simulink library "ddm"  (R2021b)
settings: Solver=VariableStepAuto  StartTime=0.0  StopTime=10.0  RelTol=1e-3
undefined symbols (not defined in the file): ADDM_FrTMTqDev_X_Nm, ADDM_RrTMTqDev_X_Nm, ENUM_ADASACCSTA_ERROR, ENUM_ADASACCSTA_OFF, ENUM_ADASACCSTA_STANDBY, ENUM_ALLOWMOV_ALLOWREADY, ENUM_APS, ENUM_BRKSTA_ERROR, ENUM_BRKSTA_OFF, ENUM_BRKSTA_ON, ENUM_BRKSW_INVALID, ENUM_BRKSW_OFF, ENUM_BRKSW_ON, ENUM_CHGPREACTERRSTA_OBCPRE, ENUM_DCDCFAULTSTA_ANYFAULTLV1, ENUM_DCDCFAULTSTA_ANYFAULTLV2, ENUM_DRIVETRAIN_AWD, ENUM_DRIVETRAIN_FWD, ENUM_DRIVETRAIN_RWD, ENUM_EDUDRTSTA_NORMAL, ENUM_EPBERROR_FAILED, ENUM_EPBSTA_APPLIED, ENUM_EPBSTA_RELEASED, ENUM_ESCAPSSta_APSUNAVAILABLE, ENUM_GEARACTUALPOSN_INVALID, ENUM_GEARACTUALPOSN_P, ENUM_HVBATTREADYPRE_READY, ENUM_HWRESETSTA_HWRESETING, ENUM_MCUWARN_LV0, ENUM_MCUWARN_LV1, ENUM_MCUWARN_LV2, ENUM_MCUWARN_LV3, ENUM_MCUWARN_NOERROR, ENUM_OBCFAULTSTA_ANYFAULT, ENUM_PAS_R2F2, ENUM_PDFAULT_BATTPDFAIL, ENUM_PDFAULT_DCDCDISABLE, ENUM_PDFAULT_MCUDISABLE, ENUM_PDFAULT_MCUDISCHRG, ENUM_POWERSTA_OFF, ENUM_POWERSTA_ON, ENUM_POWERSTA_READY, ENUM_POWERSTA_STANDBY, ENUM_PRESSINDI_LOW, ENUM_PUFAULT_BATTUPFAIL, ENUM_PUFAULT_DCDCENABLEFAIL, ENUM_PUFAULT_PRECHRGCHKFAIL, ENUM_PUFAULT_SAFETYCHKFAIL, ENUM_PWRSTASW_OFF, ENUM_PWRSTASW_OFFA, ENUM_PWRSTASW_OFFCHVCHRG, ENUM_PWRSTASW_OFFCLVCHRG, ENUM_PWRSTASW_ON, ENUM_PWRSTASW_ONHVCHRG, ENUM_PWRSTASW_READY, ENUM_PWRSTASW_STANDBY, ENUM_RAPSErrWarnSta_NORMAL, ENUM_RAPSErrWarnSta_RAPSERRLV1, ENUM_SHIFTCOMMAND_P, ENUM_SHIFTERERRSTA_PBUTTONFAILURE ... (+471)
libraries: hcu_lib x540, simulink x3
(part 20 of 26)

== system ddm/DDM/DDM/PMM/Fault level/Fault level 4 subsystem error1 ==
  note: Test Pass Criteria
  note: Release Condition After Failure Decision
  note: Diagnostics and Fault Handling
  note: Test Detection Criteria
  task_time_s : Inport
  VPMM_PowerSta_enum : Inport  Port=2
  VPMM_PwrStaSW_enum : Inport  Port=3
  VDDM_C3BMS6LCCFS_flg : Inport  Port=4
  VINP_BMSWarn7_flg : Inport  Port=5
  VINP_BMSWarn8_flg : Inport  Port=6
  DTC_clear_request : Inport  Port=7
  No_CAN3_BUS_OFF : Inport  Port=8
  VDDM_C3BMS6RCCFS_flg : Inport  Port=9
  VDDM_C3BMS6CSCFS_flg : Inport  Port=10
  ZoneDrMalfunLevel_enum : Inport  Port=11
  No_CAN4_BUS_OFF : Inport  Port=12
  VDDM_DrVCUNoComCFS_flg : Inport  Port=13
  ZoneFrMalfunLevel_enum : Inport  Port=14
  VDDM_FrVCUNoComCFS_flg : Inport  Port=15
  AND2 : Logic  Inputs=5  AllPortsSameDT=off  OutDataTypeStr=boolean
  AND5 : Logic  Inputs=3  AllPortsSameDT=off  OutDataTypeStr=boolean
  AND6 : Logic  Inputs=3  AllPortsSameDT=off  OutDataTypeStr=boolean
  Constant1 : Constant  Value=ENUM_PWRSTASW_OFF
  Constant12 : Constant  Value=KDDM_FaultLvDiagnosisOffSW_flg
  Constant14 : Constant  Value=ZERO_INT
  Constant18 : Constant  Value=KDDM_Lv4ErrPassTO_s
  Constant19 : Constant  Value=ENUM_POWERSTA_OFF
  Constant2 : Constant  Value=TRUE
  Constant22 : Constant  Value=FALSE
  Constant24 : Constant  Value=TRUE
  Constant25 : Constant  Value=FALSE
  Constant26 : Constant  Value=ENUM_PWRSTASW_OFF
  Constant27 : Constant  Value=FALSE
  Constant3 : Constant  Value=KDDM_Lv4ErrDetTO_s
  Constant4 : Constant  Value=KDDM_Lv4ErrPassTO_s
  Constant40 : Constant  Value=KDDM_Lv4ErrDTC_cnt
  Constant5 : Constant  Value=KDDM_Lv4ErrDTC_cnt
  Constant6 : Constant  Value=ENUM_ZONEMALFUNLV_4TH
  Constant7 : Constant  Value=ENUM_ZONEMALFUNLV_4TH
  DTC_Couter : hcu_lib/Basic_Blocks/DTC_Couter
  DTC_Info : hcu_lib/Basic_Blocks/DTC_Info
  Delay : Delay  DelayLength=1
  Equal : RelationalOperator  Operator=~=  OutDataTypeStr=boolean  RndMeth=Simplest
  Equal1 : RelationalOperator  Operator===  OutDataTypeStr=boolean  RndMeth=Simplest
  Equal2 : RelationalOperator  Operator=~=  OutDataTypeStr=boolean  RndMeth=Simplest
  Equal3 : RelationalOperator  OutDataTypeStr=boolean  RndMeth=Simplest
  Equal4 : RelationalOperator  Operator===  OutDataTypeStr=boolean  RndMeth=Simplest
  Equal8 : RelationalOperator  Operator===  OutDataTypeStr=boolean  RndMeth=Simplest
  Logical Operator21 : Logic  AllPortsSameDT=off  OutDataTypeStr=boolean
  Logical Operator6 : Logic  Operator=NOT  AllPortsSameDT=off  OutDataTypeStr=boolean
  Logical Operator8 : Logic  Operator=OR  Inputs=4  AllPortsSameDT=off  OutDataTypeStr=boolean
  NOT{,17..19,26,28} (6 alike) : Logic  Operator=NOT  AllPortsSameDT=off  OutDataTypeStr=boolean
  OR : Logic  Operator=OR  Inputs=3  AllPortsSameDT=off  OutDataTypeStr=boolean
  OR1 : Logic  Operator=OR  AllPortsSameDT=off  OutDataTypeStr=boolean
  OR2 : Logic  Operator=OR  Inputs=3  AllPortsSameDT=off  OutDataTypeStr=boolean
  Relational Operator : RelationalOperator  Operator=>  OutDataTypeStr=boolean  RndMeth=Simplest
  Switch{1,4..5,9} (4 alike) : Switch  Criteria=u2 ~= 0
  Terminator : Terminator
  Test Detection Criteria : hcu_lib/Basic_Blocks/Test Detection Criteria
  Timer1 : hcu_lib/Basic_Blocks/Timer
  VDDM_Lv4ErrCFS_flg : Outport
  VDDM_Lv4ErrDTC_raw32 : Outport  Port=2
  wires:
  Switch9/1 -> Test Detection Criteria/1
  Constant22/1 -> Switch9/1
  [VDDM_Lv4ErrCFSRls_flg] -> Switch9/2
  DTC_Info/1 -> VDDM_Lv4ErrDTC_raw32/1  "VDDM_Lv4ErrDTC_raw32"
  [VDDM_Lv4ErrPass_flg] -> DTC_Info/2
  [VDDM_Lv4ErrDet_flg] -> DTC_Info/1
  [VDDM_Lv4ErrCFS_flg] -> DTC_Info/3
  [DTC_clear_request] -> DTC_Info/4
  VDDM_FrVCUNoComCFS_flg/1 -> [VDDM_FrVCUNoComCFS_flg]
  ZoneFrMalfunLevel_enum/1 -> [ZoneFrMalfunLevel_enum]
  VDDM_DrVCUNoComCFS_flg/1 -> [VDDM_DrVCUNoComCFS_flg]
  No_CAN4_BUS_OFF/1 -> [No_CAN4_BUS_OFF]
  ZoneDrMalfunLevel_enum/1 -> [ZoneDrMalfunLevel_enum]
  VDDM_C3BMS6CSCFS_flg/1 -> [VDDM_C3BMS6CSCFS_flg]
  VDDM_C3BMS6RCCFS_flg/1 -> [VDDM_C3BMS6RCCFS_flg]
  [VDDM_Lv4ErrCFS_flg] -> VDDM_Lv4ErrCFS_flg/1
  Equal2/1 -> Switch1/2
  [VDDM_BMSFaultLv4_flg] -> OR2/1
  OR2/1 -> Switch1/1
  [VDDM_ZoneFrFaultLv4_flg] -> OR2/3
  Constant1/1 -> Equal2/2
  [VDDM_ZoneDrFaultLv4_flg] -> OR2/2
  [VPMM_PwrStaSW_enum] -> Equal2/1
  Constant2/1 -> Switch1/3
  OR/1 -> Switch5/1
  [VDDM_BMSFaultLv4_flg] -> OR/1
  [VDDM_ZoneDrFaultLv4_flg] -> OR/2
  [VDDM_ZoneFrFaultLv4_flg] -> OR/3
  AND5/1 -> [VDDM_ZoneDrFaultLv4_flg]  "VDDM_ZoneDrFaultLv4_flg"
  [VINP_BMSWarn7_flg] -> OR1/1
  [VDDM_C3BMS6CSCFS_flg] -> NOT19/1
  NOT19/1 -> AND2/5
  Constant7/1 -> Equal8/2
  NOT18/1 -> AND2/4
  [VINP_BMSWarn8_flg] -> OR1/2
  [No_CAN4_BUS_OFF] -> AND5/2
  [ZoneFrMalfunLevel_enum] -> Equal8/1
  Equal8/1 -> AND6/1
  NOT26/1 -> AND5/3
  [ZoneDrMalfunLevel_enum] -> Equal1/1
  OR1/1 -> AND2/1
  [VDDM_DrVCUNoComCFS_flg] -> NOT26/1
  AND2/1 -> [VDDM_BMSFaultLv4_flg]  "VDDM_BMSFaultLv4_flg"
  NOT17/1 -> AND2/3
  Constant6/1 -> Equal1/2
  Equal1/1 -> AND5/1
  [No_CAN4_BUS_OFF] -> AND6/2
  AND6/1 -> [VDDM_ZoneFrFaultLv4_flg]  "VDDM_ZoneFrFaultLv4_flg"
  [VDDM_FrVCUNoComCFS_flg] -> NOT28/1
  NOT28/1 -> AND6/3
  [VDDM_C3BMS6RCCFS_flg] -> NOT18/1
  [No_CAN3_BUS_OFF] -> AND2/2
  [VDDM_C3BMS6LCCFS_flg] -> NOT17/1
  Constant14/1 -> Relational Operator/2
  [VDDM_Lv4ErrCFSRls_flg] -> DTC_Couter/2
  [VDDM_Lv4ErrDet_flg] -> DTC_Couter/1
  [VDDM_Lv4ErrPass_flg] -> Logical Operator21/1
  Logical Operator21/1 -> Logical Operator8/3
  [VDDM_Lv4ErrCFS_flg] -> Delay/1
  Delay/1 -> NOT/1
  NOT/1 -> Logical Operator21/2
  Constant12/1 -> Logical Operator8/4
  Switch5/1 -> Switch9/3
  Constant3/1 -> Test Detection Criteria/4
  [task_time_s] -> Timer1/3
  No_CAN3_BUS_OFF/1 -> [No_CAN3_BUS_OFF]
  DTC_clear_request/1 -> [DTC_clear_request]
  [VPMM_PwrStaSW_enum] -> Equal/1
  [VPMM_PowerSta_enum] -> Equal4/1
  Constant4/1 -> Timer1/4
  Constant19/1 -> Equal4/2
  Constant25/1 -> Switch4/3
  Test Detection Criteria/1 -> [VDDM_Lv4ErrDet_flg]  "VDDM_Lv4ErrDet_flg"
  Constant27/1 -> Switch5/3
  Switch4/1 -> [VDDM_Lv4ErrCFSRls_flg]  "VDDM_Lv4ErrCFSRls_flg"
  Logical Operator8/1 -> Switch4/2
  Switch1/1 -> Timer1/2, Logical Operator6/1
  Equal/1 -> Switch5/2
  Constant24/1 -> Switch4/1
  Relational Operator/1 -> Terminator/1  "VDDM_Lv4ErrDFS_flg"
  DTC_Couter/1 -> [VDDM_Lv4ErrCFS_flg]  "VDDM_Lv4ErrCFS_flg"
  Constant18/1 -> Equal3/2
  Constant26/1 -> Equal/2
  Timer1/1 -> Equal3/1
  [DTC_clear_request] -> Logical Operator8/2
  Equal4/1 -> Logical Operator8/1
  Constant40/1 -> Test Detection Criteria/3
  DTC_Couter/2 -> Relational Operator/1  "VDDM_Lv4ErrDTC_cnt"
  [task_time_s] -> Test Detection Criteria/2
  Logical Operator6/1 -> Timer1/1
  Constant5/1 -> DTC_Couter/3
  Equal3/1 -> [VDDM_Lv4ErrPass_flg]  "VDDM_Lv4ErrPass_flg"
  VDDM_C3BMS6LCCFS_flg/1 -> [VDDM_C3BMS6LCCFS_flg]
  VINP_BMSWarn7_flg/1 -> [VINP_BMSWarn7_flg]
  task_time_s/1 -> [task_time_s]
  VPMM_PwrStaSW_enum/1 -> [VPMM_PwrStaSW_enum]
  VPMM_PowerSta_enum/1 -> [VPMM_PowerSta_enum]
  VINP_BMSWarn8_flg/1 -> [VINP_BMSWarn8_flg]

== system ddm/DDM/DDM/PMM/LV/Initial LV battery voltage too low ==
  note: Test Detection Criteria
  note: Test Pass Criteria
  note: Release Condition After Decision
  note: Diagnostics and Fault Handling
  task_time_s : Inport
  VPMM_PowerSta_enum : Inport  Port=2
  VPMM_PwrStaSW_enum : Inport  Port=3
  VDDM_AuxBatVolt_V : Inport  Port=4
  VINP_CANMsgValidBMS5_flg : Inport  Port=5
  DTC_clear_request : Inport  Port=6
  Constant1 : Constant  Value=ENUM_PWRSTASW_OFF
  Constant12 : Constant  Value=ENUM_POWERSTA_STANDBY
  Constant13 : Constant  Value=ZERO_INT
  Constant17 : Constant  Value=KDDM_IniLVLoDTC_cnt
  Constant2 : Constant  Value=ENUM_PWRSTASW_OFF
  Constant22 : Constant  Value=KDDM_IniLVLoDetTO_s
  Constant23 : Constant  Value=FALSE
  Constant26 : Constant  Value=ENUM_PWRSTASW_STANDBY
  Constant27 : Constant  Value=FALSE
  Constant28 : Constant  Value=KDDM_IniLVLoPassTO_s
  Constant29 : Constant  Value=KDDM_IniLVLoPassTO_s
  Constant3 : Constant  Value=ENUM_PWRSTASW_STANDBY
  Constant30 : Constant  Value=KDDM_IniLVLoDTC_cnt
  Constant32 : Constant  Value=KDDM_LVDiagnosisOffSW_flg
  Constant33 : Constant  Value=ENUM_POWERSTA_OFF
  Constant34 : Constant  Value=KDDM_IniLVLoThd_mv
  Constant4 : Constant  Value=FALSE
  Constant5 : Constant  Value=KDDM_IniLVLoThd_mv
  DTC_Couter1 : hcu_lib/Basic_Blocks/DTC_Couter
  DTC_Info : hcu_lib/Basic_Blocks/DTC_Info
  Equal{1..2,4,11..12,14} (6 alike) : RelationalOperator  Operator===  OutDataTypeStr=boolean  RndMeth=Simplest
  Equal10 : RelationalOperator  OutDataTypeStr=boolean  RndMeth=Simplest
  Equal13 : RelationalOperator  Operator=<=  OutDataTypeStr=boolean  RndMeth=Simplest
  Equal3 : RelationalOperator  Operator=<=  OutDataTypeStr=boolean  RndMeth=Simplest
  Gain1 : Gain  Gain=1000
  Gain3 : Gain  Gain=1000
  Logical Operator : Logic  Operator=OR  AllPortsSameDT=off  OutDataTypeStr=boolean
  Logical Operator1 : Logic  Operator=OR  AllPortsSameDT=off  OutDataTypeStr=boolean
  Logical Operator14 : Logic  Operator=OR  Inputs=4  AllPortsSameDT=off  OutDataTypeStr=boolean
  Logical Operator16 : Logic  AllPortsSameDT=off  OutDataTypeStr=boolean
  Logical Operator17 : Logic  Operator=NOT  AllPortsSameDT=off  OutDataTypeStr=boolean
  Logical Operator2 : Logic  AllPortsSameDT=off  OutDataTypeStr=boolean
  Logical Operator9 : Logic  AllPortsSameDT=off  OutDataTypeStr=boolean
  Relational Operator1 : RelationalOperator  Operator=>  OutDataTypeStr=boolean  RndMeth=Simplest
  Switch1 : Switch  Criteria=u2 ~= 0
  Switch2 : Switch  Criteria=u2 ~= 0
  Switch7 : Switch  Criteria=u2 ~= 0
  Terminator : Terminator
  Test Detection Criteria1 : hcu_lib/Basic_Blocks/Test Detection Criteria
  Timer2 : hcu_lib/Basic_Blocks/Timer
  Unit Delay1 : UnitDelay  SampleTime=-1  HasFrameUpgradeWarning=on
  VDDM_IniLVLoDTC_raw32 : Outport
  VDDM_IniLVLoCFS_flg : Outport  Port=2
  wires:
  [VDDM_IniLVLoCFS_flg] -> VDDM_IniLVLoCFS_flg/1
  [VDDM_IniLVLoPass_flg] -> Logical Operator14/3
  Logical Operator9/1 -> Switch1/2
  Constant26/1 -> Equal14/1
  Equal13/1 -> Switch1/1
  Gain3/1 -> Equal13/1
  [VDDM_AuxBatVolt_V] -> Gain3/1
  Constant34/1 -> Equal13/2
  DTC_Couter1/2 -> Relational Operator1/1  "VDDM_IniLVLoDTC_cnt"
  Constant28/1 -> Timer2/4
  DTC_Couter1/1 -> [VDDM_IniLVLoCFS_flg]  "VDDM_IniLVLoCFS_flg"
  [VDDM_IniLVLoDet_flg] -> DTC_Couter1/1
  Logical Operator16/1 -> Logical Operator14/1
  Unit Delay1/1 -> Equal11/1
  [DTC_clear_request] -> Logical Operator14/2
  Constant33/1 -> Equal11/2
  Equal11/1 -> Logical Operator16/1
  Test Detection Criteria1/1 -> [VDDM_IniLVLoDet_flg]  "VDDM_IniLVLoDet_flg"
  [VPMM_PowerSta_enum] -> Equal12/1
  Switch7/1 -> Test Detection Criteria1/1
  Constant32/1 -> Logical Operator14/4
  Constant12/1 -> Equal12/2
  [task_time_s] -> Timer2/3
  Logical Operator14/1 -> [VDDM_IniLVLoCFSRls_flg]  "VDDM_IniLVLoCFSRls_flg"
  Constant17/1 -> Test Detection Criteria1/3
  [VPMM_PowerSta_enum] -> Unit Delay1/1
  Relational Operator1/1 -> Terminator/1  "VDDM_IniLVLoDFS_flg"
  Equal12/1 -> Logical Operator16/2
  [task_time_s] -> Test Detection Criteria1/2
  Switch1/1 -> Switch7/3
  Constant30/1 -> DTC_Couter1/3
  Equal10/1 -> [VDDM_IniLVLoPass_flg]  "VDDM_IniLVLoPass_flg"
  [VDDM_IniLVLoCFSRls_flg] -> Switch7/2
  Constant23/1 -> Switch7/1
  Constant22/1 -> Test Detection Criteria1/4
  Constant29/1 -> Equal10/2
  Switch2/1 -> Logical Operator17/1, Timer2/2
  Timer2/1 -> Equal10/1
  Constant27/1 -> Switch1/3
  Logical Operator17/1 -> Timer2/1
  [VDDM_IniLVLoCFSRls_flg] -> DTC_Couter1/2
  Constant13/1 -> Relational Operator1/2
  task_time_s/1 -> [task_time_s]
  VDDM_AuxBatVolt_V/1 -> [VDDM_AuxBatVolt_V]
  VPMM_PwrStaSW_enum/1 -> [VPMM_PwrStaSW_enum]
  VPMM_PowerSta_enum/1 -> [VPMM_PowerSta_enum]
  DTC_clear_request/1 -> [DTC_clear_request]
  VINP_CANMsgValidBMS5_flg/1 -> [VINP_CANMsgValidBMS5_flg]
  DTC_Info/1 -> VDDM_IniLVLoDTC_raw32/1  "VDDM_IniLVLoDTC_raw32"
  [VDDM_IniLVLoPass_flg] -> DTC_Info/2
  [VDDM_IniLVLoCFS_flg] -> DTC_Info/3
  [VDDM_IniLVLoDet_flg] -> DTC_Info/1
  [DTC_clear_request] -> DTC_Info/4
  [VINP_CANMsgValidBMS5_flg] -> Logical Operator9/2
  Constant1/1 -> Equal1/2
  Constant5/1 -> Equal3/2
  Logical Operator2/1 -> Switch2/2
  [VDDM_AuxBatVolt_V] -> Gain1/1
  Constant4/1 -> Switch2/3
  Equal3/1 -> Switch2/1
  Gain1/1 -> Equal3/1
  Logical Operator/1 -> Logical Operator9/1
  Equal14/1 -> Logical Operator/1
  Equal1/1 -> Logical Operator/2
  [VPMM_PwrStaSW_enum] -> Equal14/2, Equal1/1
  Equal4/1 -> Logical Operator1/1
  Constant2/1 -> Equal2/2
  Constant3/1 -> Equal4/1
  Logical Operator1/1 -> Logical Operator2/1
  [VPMM_PwrStaSW_enum] -> Equal4/2, Equal2/1
  Equal2/1 -> Logical Operator1/2
  [VINP_CANMsgValidBMS5_flg] -> Logical Operator2/2

== system ddm/DDM/DDM/PMM/LV/LV analog input error ==
  note: Diagnostics and Fault Handling
  note: Release Condition After Decision
  note: Test Pass Criteria
  note: Test Detection Criteria
  task_time_s : Inport
  VPMM_PowerSta_enum : Inport  Port=2
  VINP_LVBattDet12V_V : Inport  Port=3
  VINP_CANMsgValidBMS5_flg : Inport  Port=4
  DTC_clear_request : Inport  Port=5
  VDDM_AuxBattVolV_V : Inport  Port=6
  VINP_VehicleType_enum : Inport  Port=7
  Abs : Abs
  Abs1 : Abs
  Add : Sum  Inputs=-+
  Add1 : Sum  Inputs=-+
  Constant : Constant  Value=eps
  Constant1 : Constant  Value=eps
  Constant12 : Constant  Value=ENUM_POWERSTA_STANDBY
  Constant13 : Constant  Value=ZERO_INT
  Constant17 : Constant  Value=KDDM_LVInErrDTC_cnt
  Constant2 : Constant  Value=FALSE
  Constant22 : Constant  Value=KDDM_LVInErrDetTO_s
  Constant23 : Constant  Value=FALSE
  Constant27 : Constant  Value=FALSE
  Constant28 : Constant  Value=KDDM_LVInErrPassTO_s
  Constant3 : Constant  Value=KDDM_LVInErr_pct
  Constant30 : Constant  Value=KDDM_LVInErrDTC_cnt
  Constant32 : Constant  Value=KDDM_LVDiagnosisOffSW_flg
  Constant33 : Constant  Value=ENUM_POWERSTA_OFF
  Constant34 : Constant  Value=KDDM_LVInErr_pct
  Constant4 : Constant  Value=KDDM_LVInErrPassTO_s
  Constant5 : Constant  Value=ENUM_VEHICLETYPE_D31L24
  Constant6 : Constant  Value=ENUM_VEHICLETYPE_D31L24
  DTC_Couter1 : hcu_lib/Basic_Blocks/DTC_Couter
  DTC_Info : hcu_lib/Basic_Blocks/DTC_Info
  Divide : Product  Inputs=*/
  Divide1 : Product  Inputs=*/
  Equal1 : RelationalOperator  OutDataTypeStr=boolean  RndMeth=Simplest
  Equal10 : RelationalOperator  OutDataTypeStr=boolean  RndMeth=Simplest
  Equal11 : RelationalOperator  Operator===  OutDataTypeStr=boolean  RndMeth=Simplest
  Equal12 : RelationalOperator  Operator===  OutDataTypeStr=boolean  RndMeth=Simplest
  Equal13 : RelationalOperator  OutDataTypeStr=boolean  RndMeth=Simplest
  Gain : Gain  Gain=100  OutDataTypeStr=single
  Gain1 : Gain  Gain=100  OutDataTypeStr=single
  Logical Operator : Logic  AllPortsSameDT=off  OutDataTypeStr=boolean
  Logical Operator1 : Logic  AllPortsSameDT=off  OutDataTypeStr=boolean
  Logical Operator14 : Logic  Operator=OR  Inputs=4  AllPortsSameDT=off  OutDataTypeStr=boolean
  Logical Operator16 : Logic  AllPortsSameDT=off  OutDataTypeStr=boolean
  Logical Operator17 : Logic  Operator=NOT  AllPortsSameDT=off  OutDataTypeStr=boolean
  Max : MinMax  Function=max  Inputs=2
  Max1 : MinMax  Function=max  Inputs=2
  Relational Operator : RelationalOperator  Operator=~=  OutDataTypeStr=boolean  RndMeth=Simplest
  Relational Operator1 : RelationalOperator  Operator=>  OutDataTypeStr=boolean  RndMeth=Simplest
  Relational Operator2 : RelationalOperator  Operator=~=  OutDataTypeStr=boolean  RndMeth=Simplest
  Switch1 : Switch  Criteria=u2 ~= 0
  Switch2 : Switch  Criteria=u2 ~= 0
  Switch7 : Switch  Criteria=u2 ~= 0
  Terminator : Terminator
  Test Detection Criteria1 : hcu_lib/Basic_Blocks/Test Detection Criteria
  Timer2 : hcu_lib/Basic_Blocks/Timer
  Unit Delay1 : UnitDelay  SampleTime=-1  HasFrameUpgradeWarning=on
  VDDM_LVInErrDTC_raw32 : Outport
  VDDM_LVInErrCFS_flg : Outport  Port=2
  wires:
  [VDDM_LVInErrCFS_flg] -> VDDM_LVInErrCFS_flg/1
  Constant2/1 -> Switch2/3
  [VDDM_AuxBattVolV_V] -> Add1/1
  Constant3/1 -> Equal1/2
  Equal1/1 -> Switch2/1
  [VINP_LVBattDet12V_V] -> Add1/2, Max1/1
  Gain1/1 -> Equal1/1
  Add1/1 -> Divide1/1
  Divide1/1 -> Abs1/1
  Abs1/1 -> Gain1/1
  Constant1/1 -> Max1/2
  Max1/1 -> Divide1/2
  Max/1 -> Divide/2
  Add/1 -> Divide/1
  Constant/1 -> Max/2
  [VINP_LVBattDet12V_V] -> Add/2, Max/1
  [VDDM_AuxBattVolV_V] -> Add/1
  Abs/1 -> Gain/1
  Divide/1 -> Abs/1
  VDDM_AuxBattVolV_V/1 -> [VDDM_AuxBattVolV_V]
  VPMM_PowerSta_enum/1 -> [VPMM_PowerSta_enum]
  VINP_LVBattDet12V_V/1 -> [VINP_LVBattDet12V_V]
  VINP_CANMsgValidBMS5_flg/1 -> [VINP_CANMsgValidBMS5_flg]
  [DTC_clear_request] -> DTC_Info/4
  DTC_clear_request/1 -> [DTC_clear_request]
  [VDDM_LVInErrCFS_flg] -> DTC_Info/3
  task_time_s/1 -> [task_time_s]
  DTC_Info/1 -> VDDM_LVInErrDTC_raw32/1  "VDDM_LVInErrDTC_raw32"
  [VDDM_LVInErrDet_flg] -> DTC_Info/1
  [VDDM_LVInErrPass_flg] -> DTC_Info/2
  Equal10/1 -> [VDDM_LVInErrPass_flg]  "VDDM_LVInErrPass_flg"
  Constant23/1 -> Switch7/1
  Constant13/1 -> Relational Operator1/2
  [VDDM_LVInErrCFSRls_flg] -> Switch7/2
  Constant34/1 -> Equal13/2
  DTC_Couter1/1 -> [VDDM_LVInErrCFS_flg]  "VDDM_LVInErrCFS_flg"
  Equal12/1 -> Logical Operator16/2
  [VDDM_LVInErrCFSRls_flg] -> DTC_Couter1/2
  [VPMM_PowerSta_enum] -> Equal12/1
  Constant12/1 -> Equal12/2
  Switch7/1 -> Test Detection Criteria1/1
  Gain/1 -> Equal13/1
  Constant33/1 -> Equal11/2
  [task_time_s] -> Timer2/3
  Constant30/1 -> DTC_Couter1/3
  Relational Operator1/1 -> Terminator/1  "VDDM_LVInErrDFS_flg"
  Constant22/1 -> Test Detection Criteria1/4
  Logical Operator14/1 -> [VDDM_LVInErrCFSRls_flg]  "VDDM_LVInErrCFSRls_flg"
  Constant27/1 -> Switch1/3
  [VDDM_LVInErrPass_flg] -> Logical Operator14/3
  [VPMM_PowerSta_enum] -> Unit Delay1/1
  Constant17/1 -> Test Detection Criteria1/3
  Unit Delay1/1 -> Equal11/1
  Constant4/1 -> Equal10/2
  Equal11/1 -> Logical Operator16/1
  [DTC_clear_request] -> Logical Operator14/2
  Equal13/1 -> Switch1/1
  [VDDM_LVInErrDet_flg] -> DTC_Couter1/1
  Logical Operator17/1 -> Timer2/1
  DTC_Couter1/2 -> Relational Operator1/1  "VDDM_LVInErrDTC_cnt"
  Logical Operator16/1 -> Logical Operator14/1
  Timer2/1 -> Equal10/1
  Test Detection Criteria1/1 -> [VDDM_LVInErrDet_flg]  "VDDM_LVInErrDet_flg"
  Switch1/1 -> Switch7/3
  Constant28/1 -> Timer2/4
  Switch2/1 -> Logical Operator17/1, Timer2/2
  Constant32/1 -> Logical Operator14/4
  [task_time_s] -> Test Detection Criteria1/2
  VINP_VehicleType_enum/1 -> [VINP_VehicleType_enum]
  [VINP_CANMsgValidBMS5_flg] -> Logical Operator/1
  Logical Operator/1 -> Switch1/2
  Relational Operator/1 -> Logical Operator/2
  [VINP_VehicleType_enum] -> Relational Operator/1
  Constant5/1 -> Relational Operator/2
  [VINP_CANMsgValidBMS5_flg] -> Logical Operator1/1
  [VINP_VehicleType_enum] -> Relational Operator2/1
  Constant6/1 -> Relational Operator2/2
  Relational Operator2/1 -> Logical Operator1/2
  Logical Operator1/1 -> Switch2/2

== system ddm/DDM/DDM/PMM/LV/LV power supply voltage too high ==
  note: Release Condition After Decision
  note: Test Detection Criteria
  note: Test Pass Criteria
  note: Diagnostics and Fault Handling
  task_time_s : Inport
  VPMM_PowerSta_enum : Inport  Port=2
  VPMM_PwrStaSW_enum : Inport  Port=3
  VDDM_AuxBatVolt_V : Inport  Port=4
  VINP_CANMsgValidBMS5_flg : Inport  Port=5
  DTC_clear_request : Inport  Port=6
  Constant28 : Constant  Value=ENUM_POWERSTA_STANDBY
  Constant29 : Constant  Value=ZERO_INT
  Constant30 : Constant  Value=KDDM_LVSupHiDTC_cnt
  Constant31 : Constant  Value=KDDM_LVSupHiDetTO_s
  Constant32 : Constant  Value=KDDM_LVSupHiPassTO_s
  Constant33 : Constant  Value=FALSE
  Constant34 : Constant  Value=ENUM_PWRSTASW_READY
  Constant35 : Constant  Value=ENUM_PWRSTASW_OFFCHVCHRG
  Constant36 : Constant  Value=ENUM_PWRSTASW_READY
  Constant37 : Constant  Value=ENUM_PWRSTASW_OFFCHVCHRG
  Constant38 : Constant  Value=ENUM_PWRSTASW_ON
  Constant39 : Constant  Value=ENUM_PWRSTASW_OFFCLVCHRG
  Constant42 : Constant  Value=KDDM_LVDiagnosisOffSW_flg
  Constant43 : Constant  Value=ENUM_POWERSTA_OFF
  Constant44 : Constant  Value=ENUM_PWRSTASW_ON
  Constant45 : Constant  Value=ENUM_PWRSTASW_ONHVCHRG
  Constant47 : Constant  Value=ENUM_PWRSTASW_OFFCLVCHRG
  Constant49 : Constant  Value=ENUM_PWRSTASW_ONHVCHRG
  Constant50 : Constant  Value=FALSE
  Constant51 : Constant  Value=KDDM_LVSupHiThd_mv
  Constant52 : Constant  Value=ENUM_PWRSTASW_OFFA
  Constant53 : Constant  Value=FALSE
  Constant54 : Constant  Value=KDDM_LVSupHiThd_mv
  Constant55 : Constant  Value=ENUM_PWRSTASW_OFFA
  Constant56 : Constant  Value=KDDM_LVSupHiPassTO_s
  Constant57 : Constant  Value=KDDM_LVSupHiDTC_cnt
  DTC_Couter1 : hcu_lib/Basic_Blocks/DTC_Couter
  DTC_Info : hcu_lib/Basic_Blocks/DTC_Info
  Delay1 : Delay  DelayLength=1
  Equal16 : RelationalOperator  OutDataTypeStr=boolean  RndMeth=Simplest
  Equal{17..24,26..29,31..32} (14 alike) : RelationalOperator  Operator===  OutDataTypeStr=boolean  RndMeth=Simplest
  Equal25 : RelationalOperator  OutDataTypeStr=boolean  RndMeth=Simplest
  Equal30 : RelationalOperator  OutDataTypeStr=boolean  RndMeth=Simplest
  Gain3 : Gain  Gain=KXX2XX
  Gain4 : Gain  Gain=KXX2XX
  Logical Operator{9..11,16} (4 alike) : Logic  AllPortsSameDT=off  OutDataTypeStr=boolean
  Logical Operator14 : Logic  Operator=OR  Inputs=4  AllPortsSameDT=off  OutDataTypeStr=boolean
  Logical Operator17 : Logic  Operator=NOT  AllPortsSameDT=off  OutDataTypeStr=boolean
  NOT1 : Logic  Operator=NOT  AllPortsSameDT=off  OutDataTypeStr=boolean
  OR2 : Logic  Operator=OR  Inputs=6  AllPortsSameDT=off  OutDataTypeStr=boolean
  OR3 : Logic  Operator=OR  Inputs=6  AllPortsSameDT=off  OutDataTypeStr=boolean
  Relational Operator1 : RelationalOperator  Operator=>  OutDataTypeStr=boolean  RndMeth=Simplest
  Switch1 : Switch  Criteria=u2 ~= 0
  Switch5 : Switch  Criteria=u2 ~= 0
  Switch7 : Switch  Criteria=u2 ~= 0
  Terminator : Terminator
  Test Detection Criteria1 : hcu_lib/Basic_Blocks/Test Detection Criteria
  Timer2 : hcu_lib/Basic_Blocks/Timer
  Unit Delay1 : UnitDelay  SampleTime=-1  HasFrameUpgradeWarning=on
  VDDM_LVSupHiDTC_raw32 : Outport
  VDDM_LVSupHiCFS_flg : Outport  Port=2
  wires:
  [VDDM_LVSupHiCFS_flg] -> VDDM_LVSupHiCFS_flg/1
  [VDDM_AuxBatVolt_V] -> Gain4/1
  Gain4/1 -> Equal30/1
  Constant54/1 -> Equal30/2
  Constant51/1 -> Equal25/2
  Gain3/1 -> Equal25/1
  [VDDM_AuxBatVolt_V] -> Gain3/1
  [VINP_CANMsgValidBMS5_flg] -> Logical Operator10/2
  Equal17/1 -> Logical Operator16/1
  Equal18/1 -> Logical Operator16/2
  Unit Delay1/1 -> Equal17/1
  DTC_Couter1/1 -> [VDDM_LVSupHiCFS_flg]  "VDDM_LVSupHiCFS_flg"
  Constant28/1 -> Equal18/2
  Equal22/1 -> OR3/1
  [VPMM_PowerSta_enum] -> Equal18/1
  Constant42/1 -> Logical Operator14/4
  [task_time_s] -> Timer2/3
  [VINP_CANMsgValidBMS5_flg] -> Logical Operator9/2
  [task_time_s] -> Test Detection Criteria1/2
  Equal16/1 -> [VDDM_LVSupHiPass_flg]  "VDDM_LVSupHiPass_flg"
  [VPMM_PowerSta_enum] -> Unit Delay1/1
  [VPMM_PwrStaSW_enum] -> Equal23/2, Equal24/1
  Constant33/1 -> Switch7/1
  Constant29/1 -> Relational Operator1/2
  DTC_Couter1/2 -> Relational Operator1/1  "VDDM_LVSupHiDTC_cnt"
  Logical Operator17/1 -> Timer2/1
  Constant45/1 -> Equal21/2
  Timer2/1 -> Equal16/1
  Equal27/1 -> OR2/3
  Logical Operator16/1 -> Logical Operator14/1
  Constant43/1 -> Equal17/2
  Switch7/1 -> Test Detection Criteria1/1
  [DTC_clear_request] -> Logical Operator14/2
  [VPMM_PwrStaSW_enum] -> Equal22/2, Equal21/1
  Logical Operator10/1 -> Switch5/2
  Constant38/1 -> Equal22/1
  Constant55/1 -> Equal31/2
  Equal26/1 -> OR2/4
  [VPMM_PwrStaSW_enum] -> Equal32/2, Equal31/1
  Constant53/1 -> Switch5/3
  Equal30/1 -> Switch5/1
  OR3/1 -> Logical Operator10/1
  Equal28/1 -> OR3/5
  Equal32/1 -> OR3/3
  Constant37/1 -> Equal28/1
  Constant36/1 -> Equal32/1
  Equal24/1 -> OR2/6
  Constant39/1 -> Equal29/2
  [VPMM_PwrStaSW_enum] -> Equal28/2, Equal29/1
  Equal29/1 -> OR3/6
  Equal21/1 -> OR3/2
  Equal31/1 -> OR3/4
  Constant30/1 -> Test Detection Criteria1/3
  Constant31/1 -> Test Detection Criteria1/4
  Logical Operator11/1 -> Logical Operator14/3
  OR2/1 -> Logical Operator9/1
  Constant35/1 -> Equal23/1
  Constant47/1 -> Equal24/2
  Equal19/1 -> OR2/2
  Constant44/1 -> Equal20/1
  Constant34/1 -> Equal27/1
  Equal23/1 -> OR2/5
  Equal25/1 -> Switch1/1
  Constant52/1 -> Equal26/2
  [VPMM_PwrStaSW_enum] -> Equal27/2, Equal26/1
  Equal20/1 -> OR2/1
  Constant49/1 -> Equal19/2
  Constant50/1 -> Switch1/3
  Logical Operator9/1 -> Switch1/2
  [VPMM_PwrStaSW_enum] -> Equal20/2, Equal19/1
  [VDDM_LVSupHiCFS_flg] -> Delay1/1
  [VDDM_LVSupHiCFSRls_flg] -> DTC_Couter1/2
  [VDDM_LVSupHiPass_flg] -> Logical Operator11/1
  [VDDM_LVSupHiDet_flg] -> DTC_Couter1/1
  Constant57/1 -> DTC_Couter1/3
  NOT1/1 -> Logical Operator11/2
  Delay1/1 -> NOT1/1
  Test Detection Criteria1/1 -> [VDDM_LVSupHiDet_flg]  "VDDM_LVSupHiDet_flg"
  Logical Operator14/1 -> [VDDM_LVSupHiCFSRls_flg]  "VDDM_LVSupHiCFSRls_flg"
  [VDDM_LVSupHiCFSRls_flg] -> Switch7/2
  Constant56/1 -> Equal16/2
  Relational Operator1/1 -> Terminator/1  "VDDM_LVSupHiDFS_flg"
  Constant32/1 -> Timer2/4
  Switch5/1 -> Timer2/2, Logical Operator17/1
  Switch1/1 -> Switch7/3
  task_time_s/1 -> [task_time_s]
  VDDM_AuxBatVolt_V/1 -> [VDDM_AuxBatVolt_V]
  DTC_clear_request/1 -> [DTC_clear_request]
  VINP_CANMsgValidBMS5_flg/1 -> [VINP_CANMsgValidBMS5_flg]
  VPMM_PowerSta_enum/1 -> [VPMM_PowerSta_enum]
  VPMM_PwrStaSW_enum/1 -> [VPMM_PwrStaSW_enum]
  DTC_Info/1 -> VDDM_LVSupHiDTC_raw32/1  "VDDM_LVSupHiDTC_raw32"
  [VDDM_LVSupHiPass_flg] -> DTC_Info/2
  [VDDM_LVSupHiCFS_flg] -> DTC_Info/3
  [VDDM_LVSupHiDet_flg] -> DTC_Info/1
  [DTC_clear_request] -> DTC_Info/4

== system ddm/DDM/DDM/PMM/LV/LV power supply voltage too low ==
  note: Diagnostics and Fault Handling
  note: Release Condition After Decision
  note: Test Pass Criteria
  note: Test Detection Criteria
  task_time_s : Inport
  VPMM_PowerSta_enum : Inport  Port=2
  VPMM_PwrStaSW_enum : Inport  Port=3
  VDDM_AuxBatVolt_V : Inport  Port=4
  VINP_CANMsgValidBMS5_flg : Inport  Port=5
  DTC_clear_request : Inport  Port=6
  Constant28 : Constant  Value=ENUM_POWERSTA_STANDBY
  Constant29 : Constant  Value=ZERO_INT
  Constant30 : Constant  Value=KDDM_LVSupLoDTC_cnt
  Constant31 : Constant  Value=KDDM_LVSupLoDetTO_s
  Constant32 : Constant  Value=KDDM_LVSupLoPassTO_s
  Constant33 : Constant  Value=FALSE
  Constant34 : Constant  Value=ENUM_PWRSTASW_READY
  Constant35 : Constant  Value=ENUM_PWRSTASW_OFFCHVCHRG
  Constant36 : Constant  Value=ENUM_PWRSTASW_READY
  Constant37 : Constant  Value=ENUM_PWRSTASW_OFFCHVCHRG
  Constant38 : Constant  Value=ENUM_PWRSTASW_ON
  Constant39 : Constant  Value=ENUM_PWRSTASW_OFFCLVCHRG
  Constant42 : Constant  Value=KDDM_LVDiagnosisOffSW_flg
  Constant43 : Constant  Value=ENUM_POWERSTA_OFF
  Constant44 : Constant  Value=ENUM_PWRSTASW_ON
  Constant45 : Constant  Value=ENUM_PWRSTASW_ONHVCHRG
  Constant47 : Constant  Value=ENUM_PWRSTASW_OFFCLVCHRG
  Constant49 : Constant  Value=ENUM_PWRSTASW_ONHVCHRG
  Constant50 : Constant  Value=FALSE
  Constant51 : Constant  Value=KDDM_LVSupLoThd_mv
  Constant52 : Constant  Value=ENUM_PWRSTASW_OFFA
  Constant53 : Constant  Value=FALSE
  Constant54 : Constant  Value=KDDM_LVSupLoThd_mv
  Constant55 : Constant  Value=ENUM_PWRSTASW_OFFA
  Constant56 : Constant  Value=KDDM_LVSupLoPassTO_s
  Constant57 : Constant  Value=KDDM_LVSupLoDTC_cnt
  DTC_Couter1 : hcu_lib/Basic_Blocks/DTC_Couter
  DTC_Info : hcu_lib/Basic_Blocks/DTC_Info
  Delay1 : Delay  DelayLength=1
  Equal16 : RelationalOperator  OutDataTypeStr=boolean  RndMeth=Simplest
  Equal{17..24,26..29,31..32} (14 alike) : RelationalOperator  Operator===  OutDataTypeStr=boolean  RndMeth=Simplest
  Equal25 : RelationalOperator  Operator=<=  OutDataTypeStr=boolean  RndMeth=Simplest
  Equal30 : RelationalOperator  Operator=<=  OutDataTypeStr=boolean  RndMeth=Simplest
  Gain3 : Gain  Gain=1000
  Gain4 : Gain  Gain=1000
  Logical Operator{9..11,16} (4 alike) : Logic  AllPortsSameDT=off  OutDataTypeStr=boolean
  Logical Operator14 : Logic  Operator=OR  Inputs=4  AllPortsSameDT=off  OutDataTypeStr=boolean
  Logical Operator17 : Logic  Operator=NOT  AllPortsSameDT=off  OutDataTypeStr=boolean
  NOT1 : Logic  Operator=NOT  AllPortsSameDT=off  OutDataTypeStr=boolean
  OR2 : Logic  Operator=OR  Inputs=6  AllPortsSameDT=off  OutDataTypeStr=boolean
  OR3 : Logic  Operator=OR  Inputs=6  AllPortsSameDT=off  OutDataTypeStr=boolean
  Relational Operator1 : RelationalOperator  Operator=>  OutDataTypeStr=boolean  RndMeth=Simplest
  Switch1 : Switch  Criteria=u2 ~= 0
  Switch5 : Switch  Criteria=u2 ~= 0
  Switch7 : Switch  Criteria=u2 ~= 0
  Terminator : Terminator
  Test Detection Criteria1 : hcu_lib/Basic_Blocks/Test Detection Criteria
  Timer2 : hcu_lib/Basic_Blocks/Timer
  Unit Delay1 : UnitDelay  SampleTime=-1  HasFrameUpgradeWarning=on
  VDDM_LVSupLoDTC_raw32 : Outport
  VDDM_LVSupLoCFS_flg : Outport  Port=2
  wires:
  [VDDM_LVSupLoCFS_flg] -> VDDM_LVSupLoCFS_flg/1
  Logical Operator11/1 -> Logical Operator14/3
  [VDDM_LVSupLoCFS_flg] -> Delay1/1
  NOT1/1 -> Logical Operator11/2
  Delay1/1 -> NOT1/1
  [VDDM_LVSupLoPass_flg] -> Logical Operator11/1
  OR3/1 -> Logical Operator10/1
  [VINP_CANMsgValidBMS5_flg] -> Logical Operator10/2
  Constant37/1 -> Equal28/1
  Equal31/1 -> OR3/4
  [VDDM_AuxBatVolt_V] -> Gain4/1
  Equal29/1 -> OR3/6
  Constant39/1 -> Equal29/2
  Equal21/1 -> OR3/2
  [VPMM_PwrStaSW_enum] -> Equal28/2, Equal29/1
  Constant54/1 -> Equal30/2
  Constant38/1 -> Equal22/1
  Equal32/1 -> OR3/3
  Constant36/1 -> Equal32/1
  Equal28/1 -> OR3/5
  Equal30/1 -> Switch5/1
  Constant53/1 -> Switch5/3
  Constant55/1 -> Equal31/2
  [VPMM_PwrStaSW_enum] -> Equal32/2, Equal31/1
  Constant45/1 -> Equal21/2
  Equal22/1 -> OR3/1
  Gain4/1 -> Equal30/1
  Logical Operator10/1 -> Switch5/2
  [VPMM_PwrStaSW_enum] -> Equal22/2, Equal21/1
  Switch1/1 -> Switch7/3
  [VPMM_PwrStaSW_enum] -> Equal20/2, Equal19/1
  Constant50/1 -> Switch1/3
  Logical Operator9/1 -> Switch1/2
  Constant49/1 -> Equal19/2
  Gain3/1 -> Equal25/1
  Equal20/1 -> OR2/1
  [VPMM_PwrStaSW_enum] -> Equal27/2, Equal26/1
  Constant52/1 -> Equal26/2
  Equal25/1 -> Switch1/1
  Equal23/1 -> OR2/5
  Equal27/1 -> OR2/3
  Constant34/1 -> Equal27/1
  Constant44/1 -> Equal20/1
  Equal19/1 -> OR2/2
  Constant51/1 -> Equal25/2
  [VPMM_PwrStaSW_enum] -> Equal23/2, Equal24/1
  Constant47/1 -> Equal24/2
  [VDDM_AuxBatVolt_V] -> Gain3/1
  Constant35/1 -> Equal23/1
  Equal24/1 -> OR2/6
  Equal26/1 -> OR2/4
  OR2/1 -> Logical Operator9/1
  [VINP_CANMsgValidBMS5_flg] -> Logical Operator9/2
  [task_time_s] -> Test Detection Criteria1/2
  Switch5/1 -> Timer2/2, Logical Operator17/1
  Equal17/1 -> Logical Operator16/1
  [VDDM_LVSupLoCFSRls_flg] -> Switch7/2
  Relational Operator1/1 -> Terminator/1  "VDDM_LVSupLoDFS_flg"
  DTC_Couter1/1 -> [VDDM_LVSupLoCFS_flg]  "VDDM_LVSupLoCFS_flg"
  [VDDM_LVSupLoDet_flg] -> DTC_Couter1/1
  Equal18/1 -> Logical Operator16/2
  [VPMM_PowerSta_enum] -> Unit Delay1/1
  [VDDM_LVSupLoCFSRls_flg] -> DTC_Couter1/2
  [task_time_s] -> Timer2/3
  Constant28/1 -> Equal18/2
  Constant42/1 -> Logical Operator14/4
  [VPMM_PowerSta_enum] -> Equal18/1
  [DTC_clear_request] -> Logical Operator14/2
  Switch7/1 -> Test Detection Criteria1/1
  Constant56/1 -> Equal16/2
  Constant57/1 -> DTC_Couter1/3
  Constant43/1 -> Equal17/2
  Constant30/1 -> Test Detection Criteria1/3
  Constant31/1 -> Test Detection Criteria1/4
  Test Detection Criteria1/1 -> [VDDM_LVSupLoDet_flg]  "VDDM_LVSupLoDet_flg"
  Logical Operator16/1 -> Logical Operator14/1
  Unit Delay1/1 -> Equal17/1
  DTC_Couter1/2 -> Relational Operator1/1  "VDDM_LVSupLoDTC_cnt"
  Logical Operator17/1 -> Timer2/1
  Timer2/1 -> Equal16/1
  Equal16/1 -> [VDDM_LVSupLoPass_flg]  "VDDM_LVSupLoPass_flg"
  Constant33/1 -> Switch7/1
  Constant29/1 -> Relational Operator1/2
  Constant32/1 -> Timer2/4
  Logical Operator14/1 -> [VDDM_LVSupLoCFSRls_flg]  "VDDM_LVSupLoCFSRls_flg"
  task_time_s/1 -> [task_time_s]
  VDDM_AuxBatVolt_V/1 -> [VDDM_AuxBatVolt_V]
  VPMM_PwrStaSW_enum/1 -> [VPMM_PwrStaSW_enum]
  VPMM_PowerSta_enum/1 -> [VPMM_PowerSta_enum]
  DTC_clear_request/1 -> [DTC_clear_request]
  VINP_CANMsgValidBMS5_flg/1 -> [VINP_CANMsgValidBMS5_flg]
  DTC_Info/1 -> VDDM_LVSupLoDTC_raw32/1  "VDDM_LVSupLoDTC_raw32"
  [VDDM_LVSupLoPass_flg] -> DTC_Info/2
  [VDDM_LVSupLoCFS_flg] -> DTC_Info/3
  [VDDM_LVSupLoDet_flg] -> DTC_Info/1
  [DTC_clear_request] -> DTC_Info/4

== system ddm/DDM/DDM/PMM/SW failure/Driver seat switch failure ==
  note: Diagnostics and Fault Handling
  note: Release Condition After Decision
  note: Test Pass Criteria
  note: Test Detection Criteria
  task_time_s : Inport
  VPMM_PowerSta_enum : Inport  Port=2
  VPMM_PwrStaSW_enum : Inport  Port=3
  VINP_DrStSW : Inport  Port=4
  DTC_clear_request : Inport  Port=5
  Constant1 : Constant  Value=KDDM_DrStSWDTC_cnt
  Constant12 : Constant  Value=ENUM_POWERSTA_STANDBY
  Constant13 : Constant  Value=ZERO_INT
  Constant15 : Constant  Value=KDDM_DrStSWDetTO_s
  Constant16 : Constant  Value=KDDM_DrStSWDTC_cnt
  Constant17 : Constant  Value=KDDM_DrStSWPassTO_s
  Constant18 : Constant  Value=FALSE
  Constant19 : Constant  Value=ENUM_PWRSTASW_OFF
  Constant20 : Constant  Value=KDDM_DrStSWPassTO_s
  Constant21 : Constant  Value=ZERO_INT
  Constant22 : Constant  Value=ENUM_PWRSTASW_OFF
  Constant23 : Constant  Value=TRUE
  Constant24 : Constant  Value=KDDM_DrStSWPassTO_s
  Constant26 : Constant  Value=ONE_INT
  Constant27 : Constant  Value=KDDM_DrStSW_s
  Constant32 : Constant  Value=KDDM_SWFailDiagnosisOffSW_flg
  Constant33 : Constant  Value=ENUM_POWERSTA_OFF
  Constant8 : Constant  Value=ZERO_FLOAT
  DTC_Couter2 : hcu_lib/Basic_Blocks/DTC_Couter
  DTC_Info : hcu_lib/Basic_Blocks/DTC_Info
  Data Type Conversion11 : DataTypeConversion
  Data Type Conversion12 : DataTypeConversion  OutDataTypeStr=boolean
  Equal1 : RelationalOperator  Operator=~=  OutDataTypeStr=boolean  RndMeth=Simplest
  Equal11 : RelationalOperator  Operator===  OutDataTypeStr=boolean  RndMeth=Simplest
  Equal12 : RelationalOperator  Operator===  OutDataTypeStr=boolean  RndMeth=Simplest
  Equal2 : RelationalOperator  Operator=~=  OutDataTypeStr=boolean  RndMeth=Simplest
  Equal3 : RelationalOperator  Operator=~=  OutDataTypeStr=boolean  RndMeth=Simplest
  Equal5 : RelationalOperator  OutDataTypeStr=boolean  RndMeth=Simplest
  Logical Operator14 : Logic  Operator=OR  Inputs=4  AllPortsSameDT=off  OutDataTypeStr=boolean
  Logical Operator16 : Logic  AllPortsSameDT=off  OutDataTypeStr=boolean
  Logical Operator4 : Logic  Operator=NOT  AllPortsSameDT=off  OutDataTypeStr=boolean
  Logical Operator5 : Logic  Operator=NOT  AllPortsSameDT=off  OutDataTypeStr=boolean
  Logical Operator6 : Logic  AllPortsSameDT=off  OutDataTypeStr=boolean
  Logical Operator7 : Logic  Operator=NOT  AllPortsSameDT=off  OutDataTypeStr=boolean
  Relational Operator1 : RelationalOperator  Operator=>  OutDataTypeStr=boolean  RndMeth=Simplest
  Relational Operator3 : RelationalOperator  Operator=>  OutDataTypeStr=boolean  RndMeth=Simplest
  Relational Operator4 : RelationalOperator  Operator=<=  OutDataTypeStr=boolean  RndMeth=Simplest
  SR_Latch1 : hcu_lib/Basic_Blocks/SR_Latch
  Subsystem : Subsystem
  Switch10 : Switch  Criteria=u2 ~= 0
  Switch14 : Switch  Criteria=u2 ~= 0
  Switch5 : Switch  Criteria=u2 ~= 0
  Terminator : Terminator
  Test Detection Criteria2 : hcu_lib/Basic_Blocks/Test Detection Criteria
  Timer : hcu_lib/Basic_Blocks/Test Detection Criteria/Timer
  Timer1 : hcu_lib/Basic_Blocks/Timer
  Unit Delay : UnitDelay  SampleTime=-1  HasFrameUpgradeWarning=on
  Unit Delay1 : UnitDelay  SampleTime=-1  HasFrameUpgradeWarning=on
  Unit Delay7 : UnitDelay  SampleTime=-1  HasFrameUpgradeWarning=on
  VDDM_DrStSWDTC_raw32 : Outport
  VDDM_DrStSWCFS_flg : Outport  Port=2
  wires:
  [VDDM_DrStSWCFS_flg] -> VDDM_DrStSWCFS_flg/1
  Equal11/1 -> Logical Operator16/1
  Relational Operator1/1 -> Terminator/1  "VDDM_DrStSWDFS_flg"
  DTC_Couter2/1 -> [VDDM_DrStSWCFS_flg]  "VDDM_DrStSWCFS_flg"
  [VDDM_DrStSWDet_flg] -> DTC_Couter2/1
  [VDDM_DrStSWPass_flg] -> Logical Operator14/3
  Equal12/1 -> Logical Operator16/2
  [VPMM_PowerSta_enum] -> Unit Delay1/1
  [VDDM_DrStSWCFSRls_flg] -> DTC_Couter2/2
  Constant12/1 -> Equal12/2
  Constant32/1 -> Logical Operator14/4
  [VPMM_PowerSta_enum] -> Equal12/1
  [DTC_clear_request] -> Logical Operator14/2
  Constant1/1 -> DTC_Couter2/3
  Constant33/1 -> Equal11/2
  Logical Operator16/1 -> Logical Operator14/1
  Unit Delay1/1 -> Equal11/1
  DTC_Couter2/2 -> Relational Operator1/1  "VDDM_DrStSWDTC_cnt"
  Constant13/1 -> Relational Operator1/2
  Logical Operator14/1 -> [VDDM_DrStSWCFSRls_flg]  "VDDM_DrStSWCFSRls_flg"
  [task_time_s] -> Timer/3
  Constant27/1 -> Relational Operator4/2
  Relational Operator3/1 -> Unit Delay7/1, Equal2/2
  Constant24/1 -> Timer1/4
  [VINP_DrStSWGPIO_flg] -> Relational Operator3/1
  Unit Delay7/1 -> Equal2/1
  Constant8/1 -> Relational Operator3/2
  [VPMM_PwrStaSW_enum] -> Equal3/1
  [task_time_s] -> Timer1/3
  Timer1/1 -> Equal5/1
  Constant19/1 -> Equal3/2
  Constant23/1 -> Switch10/3
  Data Type Conversion12/1 -> Test Detection Criteria2/1
  Logical Operator6/1 -> Switch14/1, [DrStSWFault_flg]
  Unit Delay/1 -> Subsystem/1(In1)
  Equal5/1 -> [VDDM_DrStSWPass_flg]  "VDDM_DrStSWPass_flg"
  Switch10/1 -> Timer1/2, Logical Operator7/1
  Equal3/1 -> Switch10/2
  Logical Operator7/1 -> Timer1/1
  [task_time_s] -> Test Detection Criteria2/2
  Relational Operator4/1 -> Logical Operator6/2
  Constant16/1 -> Test Detection Criteria2/3
  [VDDM_DrStSWChange_flg] -> SR_Latch1/2
  Subsystem/1(Fault_flg) -> Logical Operator6/1
  Logical Operator4/1 -> Timer/2
  Equal2/1 -> [VDDM_DrStSWChange_flg]
  Data Type Conversion11/1 -> Test Detection Criteria2/4
  Equal1/1 -> Switch14/2
  Constant21/1 -> Switch14/3
  Constant22/1 -> Equal1/2
  [VPMM_PwrStaSW_enum] -> Equal1/1
  Test Detection Criteria2/1 -> [VDDM_DrStSWDet_flg]  "VDDM_DrStSWDet_flg"
  Switch14/1 -> Switch5/3
  [DrStSWFault_flg] -> Switch10/1
  Constant20/1 -> Equal5/2
  Logical Operator5/1 -> Subsystem/Trigger
  Constant26/1 -> SR_Latch1/1
  Constant15/1 -> Data Type Conversion11/1
  Constant18/1 -> Switch5/1
  Switch5/1 -> Data Type Conversion12/1
  [VDDM_DrStSWCFSRls_flg] -> Switch5/2
  Timer/1 -> Unit Delay/1, Relational Operator4/1
  Constant17/1 -> Timer/4
  SR_Latch1/1 -> Timer/1, Logical Operator4/1, Logical Operator5/1
  DTC_clear_request/1 -> [DTC_clear_request]
  VINP_DrStSW/1 -> [VINP_DrStSWGPIO_flg]
  task_time_s/1 -> [task_time_s]
  VPMM_PowerSta_enum/1 -> [VPMM_PowerSta_enum]
  VPMM_PwrStaSW_enum/1 -> [VPMM_PwrStaSW_enum]
  DTC_Info/1 -> VDDM_DrStSWDTC_raw32/1  "VDDM_DrStSWDTC_raw32"
  [VDDM_DrStSWPass_flg] -> DTC_Info/2
  [VDDM_DrStSWCFS_flg] -> DTC_Info/3
  [VDDM_DrStSWDet_flg] -> DTC_Info/1
  [DTC_clear_request] -> DTC_Info/4

== system ddm/DDM/DDM/PMM/SW failure/FL Door switch failure ==
  note: Diagnostics and Fault Handling
  note: Release Condition After Decision
  note: Test Detection Criteria
  note: Test Pass Criteria
  task_time_s : Inport
  VPMM_PowerSta_enum : Inport  Port=2
  VPMM_PwrStaSW_enum : Inport  Port=3
  VINP_FLAJARSW : Inport  Port=4
  DTC_clear_request : Inport  Port=5
  Constant1 : Constant  Value=KDDM_FLDoorSWDTC_cnt
  Constant11 : Constant  Value=KDDM_FLDoorSWPassTO_s
  Constant12 : Constant  Value=ENUM_POWERSTA_STANDBY
  Constant13 : Constant  Value=ZERO_INT
  Constant15 : Constant  Value=KDDM_FLDoorSWPassTO_s
  Constant16 : Constant  Value=KDDM_FLDoorSWDetTO_s
  Constant17 : Constant  Value=KDDM_FLDoorSW_s
  Constant18 : Constant  Value=FALSE
  Constant19 : Constant  Value=ENUM_PWRSTASW_OFF
  Constant2 : Constant  Value=KDDM_SWFailDiagnosisOffSW_flg
  Constant21 : Constant  Value=ZERO_INT
  Constant22 : Constant  Value=ENUM_PWRSTASW_OFF
  Constant23 : Constant  Value=TRUE
  Constant24 : Constant  Value=KDDM_FLDoorSWPassTO_s
  Constant25 : Constant  Value=KDDM_FLDoorSWDTC_cnt
  Constant26 : Constant  Value=ONE_INT
  Constant3 : Constant  Value=FALSE
  Constant32 : Constant  Value=ZERO_FLOAT
  Constant33 : Constant  Value=ENUM_POWERSTA_OFF
  Constant4 : Constant  Value=TRUE
  DTC_Couter2 : hcu_lib/Basic_Blocks/DTC_Couter
  DTC_Info : hcu_lib/Basic_Blocks/DTC_Info
  Data Type Conversion12 : DataTypeConversion  OutDataTypeStr=boolean
  Data Type Conversion14 : DataTypeConversion  OutDataTypeStr=boolean
  Data Type Conversion7 : DataTypeConversion
  Equal1 : RelationalOperator  Operator=~=  OutDataTypeStr=boolean  RndMeth=Simplest
  Equal11 : RelationalOperator  Operator===  OutDataTypeStr=boolean  RndMeth=Simplest
  Equal12 : RelationalOperator  Operator===  OutDataTypeStr=boolean  RndMeth=Simplest
  Equal3 : RelationalOperator  Operator=~=  OutDataTypeStr=boolean  RndMeth=Simplest
  Equal4 : RelationalOperator  Operator=~=  OutDataTypeStr=boolean  RndMeth=Simplest
  Equal5 : RelationalOperator  OutDataTypeStr=boolean  RndMeth=Simplest
  Logical Operator14 : Logic  Operator=OR  Inputs=4  AllPortsSameDT=off  OutDataTypeStr=boolean
  Logical Operator16 : Logic  AllPortsSameDT=off  OutDataTypeStr=boolean
  Logical Operator4 : Logic  Operator=NOT  AllPortsSameDT=off  OutDataTypeStr=boolean
  Logical Operator5 : Logic  Operator=NOT  AllPortsSameDT=off  OutDataTypeStr=boolean
  Logical Operator6 : Logic  AllPortsSameDT=off  OutDataTypeStr=boolean
  Logical Operator7 : Logic  Operator=NOT  AllPortsSameDT=off  OutDataTypeStr=boolean
  Relational Operator1 : RelationalOperator  Operator=>  OutDataTypeStr=boolean  RndMeth=Simplest
  Relational Operator4 : RelationalOperator  Operator=<=  OutDataTypeStr=boolean  RndMeth=Simplest
  Relational Operator5 : RelationalOperator  Operator=>  OutDataTypeStr=boolean  RndMeth=Simplest
  SR_Latch1 : hcu_lib/Basic_Blocks/SR_Latch
  Subsystem : Subsystem  AncestorBlock=ddm1/DDM/DDM/PMM/SW failure/Driver seat switch failure/Subsystem
  Switch{1,5,10,14} (4 alike) : Switch  Criteria=u2 ~= 0
  Terminator : Terminator
  Test Detection Criteria2 : hcu_lib/Basic_Blocks/Test Detection Criteria
  Timer : hcu_lib/Basic_Blocks/Test Detection Criteria/Timer
  Timer1 : hcu_lib/Basic_Blocks/Timer
  Unit Delay : UnitDelay  SampleTime=-1  HasFrameUpgradeWarning=on
  Unit Delay1 : UnitDelay  SampleTime=-1  HasFrameUpgradeWarning=on
  Unit Delay9 : UnitDelay  SampleTime=-1  HasFrameUpgradeWarning=on
  VDDM_FLDoorSWDTC_raw32 : Outport
  VDDM_VCUFLDoorSta_flg : Outport  Port=2
  VDDM_FLDoorSWCFS_flg : Outport  Port=3
  wires:
  Switch1/1 -> VDDM_VCUFLDoorSta_flg/1  "VDDM_VCUFLDoorSta_flg"
  Constant4/1 -> Switch1/1
  Constant3/1 -> Switch1/3
  [VDDM_FLDoorSWCFS_flg] -> VDDM_FLDoorSWCFS_flg/1, Switch1/2
  Constant12/1 -> Equal12/2
  [VDDM_FLDoorSWPass_flg] -> Logical Operator14/3
  Constant33/1 -> Equal11/2
  Relational Operator1/1 -> Terminator/1  "VDDM_FLDoorSWDFS_flg"
  Unit Delay1/1 -> Equal11/1
  Constant13/1 -> Relational Operator1/2
  [DTC_clear_request] -> Logical Operator14/2
  DTC_Couter2/2 -> Relational Operator1/1  "VDDM_FLDoorSWDTC_cnt"
  Logical Operator16/1 -> Logical Operator14/1
  [VPMM_PowerSta_enum] -> Equal12/1
  Logical Operator14/1 -> [VDDM_FLDoorSWCFSRls_flg]  "VDDM_FLDoorSWCFSRls_flg"
  Constant2/1 -> Logical Operator14/4
  [VPMM_PowerSta_enum] -> Unit Delay1/1
  Equal12/1 -> Logical Operator16/2
  Equal11/1 -> Logical Operator16/1
  DTC_Couter2/1 -> [VDDM_FLDoorSWCFS_flg]  "VDDM_FLDoorSWCFS_flg"
  [VDDM_FLDoorSWCFSRls_flg] -> DTC_Couter2/2
  Constant1/1 -> DTC_Couter2/3
  [VDDM_FLDoorSWDet_flg] -> DTC_Couter2/1
  Test Detection Criteria2/1 -> [VDDM_FLDoorSWDet_flg]  "VDDM_FLDoorSWDet_flg"
  [VINP_FL_AJAR_SW] -> Relational Operator5/1
  Unit Delay9/1 -> Data Type Conversion14/1
  Relational Operator5/1 -> Equal4/2, Unit Delay9/1
  Constant32/1 -> Relational Operator5/2
  Equal4/1 -> [VDDM_FLDoorSWChange_flg]
  Data Type Conversion14/1 -> Equal4/1
  Constant22/1 -> Equal1/2
  [task_time_s] -> Timer/3
  [VPMM_PwrStaSW_enum] -> Equal1/1
  Constant21/1 -> Switch14/3
  [VDDM_FLDoorSWChange_flg] -> SR_Latch1/2
  [task_time_s] -> Test Detection Criteria2/2
  Constant25/1 -> Test Detection Criteria2/3
  Constant23/1 -> Switch10/3
  Data Type Conversion7/1 -> Test Detection Criteria2/4
  Equal1/1 -> Switch14/2
  Logical Operator4/1 -> Timer/2
  [FLDoorSWFault_flg] -> Switch10/1
  [task_time_s] -> Timer1/3
  Subsystem/1(Fault_flg) -> Logical Operator6/1
  [VPMM_PwrStaSW_enum] -> Equal3/1
  Logical Operator7/1 -> Timer1/1
  Constant24/1 -> Equal5/2
  Relational Operator4/1 -> Logical Operator6/2
  Constant15/1 -> Timer1/4
  Equal3/1 -> Switch10/2
  Equal5/1 -> [VDDM_FLDoorSWPass_flg]
  Switch10/1 -> Timer1/2, Logical Operator7/1
  Logical Operator5/1 -> Subsystem/Trigger
  Timer/1 -> Unit Delay/1, Relational Operator4/1
  Unit Delay/1 -> Subsystem/1(In1)
  Logical Operator6/1 -> Switch14/1, [FLDoorSWFault_flg]
  Data Type Conversion12/1 -> Test Detection Criteria2/1
  Constant19/1 -> Equal3/2
  Timer1/1 -> Equal5/1
  [VDDM_FLDoorSWCFSRls_flg] -> Switch5/2
  Constant11/1 -> Timer/4
  Constant17/1 -> Relational Operator4/2
  SR_Latch1/1 -> Timer/1, Logical Operator4/1, Logical Operator5/1
  Constant18/1 -> Switch5/1
  Constant16/1 -> Data Type Conversion7/1
  Switch5/1 -> Data Type Conversion12/1
  Constant26/1 -> SR_Latch1/1
  Switch14/1 -> Switch5/3
  task_time_s/1 -> [task_time_s]
  VINP_FLAJARSW/1 -> [VINP_FL_AJAR_SW]
  DTC_clear_request/1 -> [DTC_clear_request]
  VPMM_PwrStaSW_enum/1 -> [VPMM_PwrStaSW_enum]
  VPMM_PowerSta_enum/1 -> [VPMM_PowerSta_enum]
  DTC_Info/1 -> VDDM_FLDoorSWDTC_raw32/1  "VDDM_FLDoorSWDTC_raw32"
  [VDDM_FLDoorSWPass_flg] -> DTC_Info/2
  [VDDM_FLDoorSWCFS_flg] -> DTC_Info/3
  [VDDM_FLDoorSWDet_flg] -> DTC_Info/1
  [DTC_clear_request] -> DTC_Info/4
